simulink model "Propergation_Test"  (R2025b)
settings: Solver=FixedStepAuto  StartTime=0.0  StopTime=inf  RelTol=1e-3
undefined symbols (not defined in the file): bus_b, bus_c
settings Model: SimulationMode=external  Creator=kueh_js  LastModifiedBy=kueh_js
settings OptimizationCC: OptimizeBlockIOStorage=off  EnhancedBackFolding=on  PassReuseOutputArgsThreshold=0.0  ZeroExternalMemoryAtStartup=off  ZeroInternalMemoryAtStartup=off  OptimizeBlockOrder=speed  DifferentSizesBufferReuse=on
settings DebuggingCC: ParameterTunabilityLossMsg=error
settings HardwareCC: ProdBitPerLong=64.0  ProdHWDeviceType=Intel->x86-64 (Linux 64)
settings SFSimCC: MATLABDynamicMemAlloc=off  SimTargetLang=C++  SimDLTargetLibrary=mkl-dnn
settings RTWCC: GenCodeOnly=on  Toolchain=GNU gcc/g++ | gmake (64-bit Linux)  TargetLang=C++
settings CodeAppCC: ForceParamTrailComments=on  OperatorAnnotations=on  MATLABSourceComments=on
settings GRTTargetCC: TargetLangStandard=C++20 (ISO)  MatFileLogging=off  CodeInterfacePackaging=C++ class

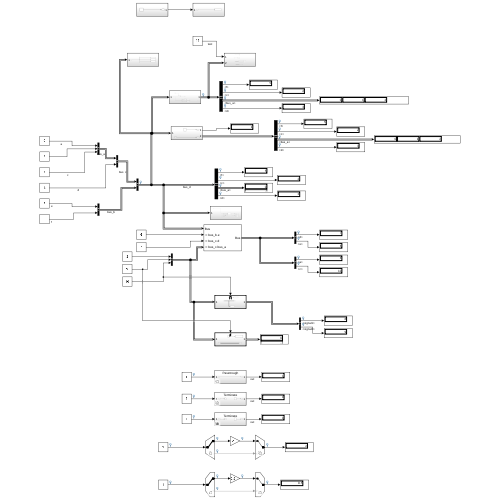
[thumbnail: Simulink's stored preview of the top-level diagram]
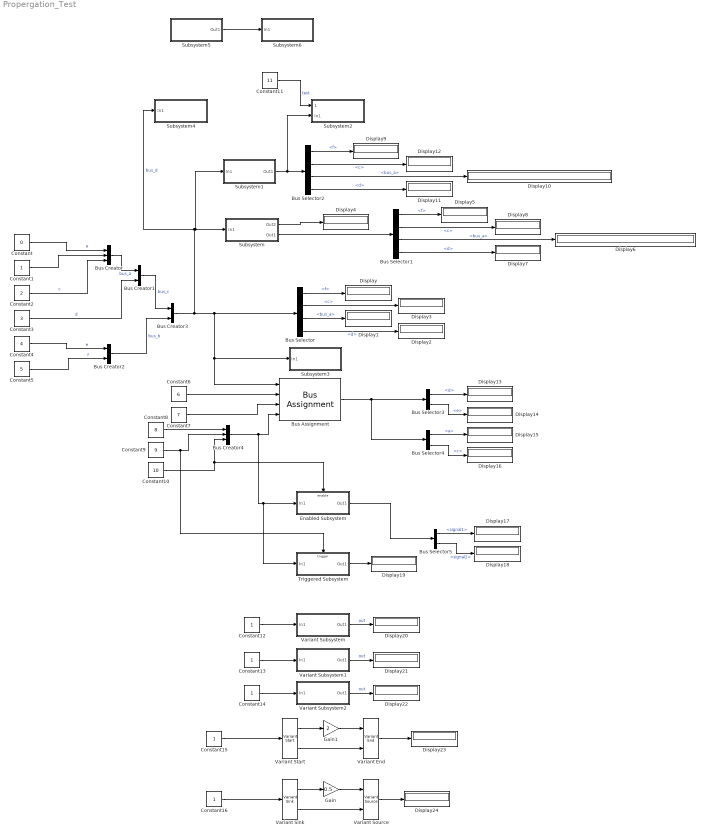
== system Propergation_Test ==
  Bus Assignment : BusAssignment  AssignedSignals=bus_b.e,bus_c.d,bus_c.bus_a
  Bus Creator : BusCreator  Inputs=3
  Bus Creator1 : BusCreator  Inputs=2
  Bus Creator2 : BusCreator  Inputs=2
  Bus Creator3 : BusCreator  Inputs=2
  Bus Creator4 : BusCreator  Inputs=3
  Bus Selector : BusSelector  OutputSignals=bus_b.f,bus_c.bus_a.c,bus_c.bus_a,bus_c.d
  Bus Selector1 : BusSelector  OutputSignals=bus_b.f,bus_c.bus_a.c,bus_c.bus_a,bus_c.d
  Bus Selector2 : BusSelector  OutputSignals=bus_d.bus_b.f,bus_d.bus_c.bus_a.c,bus_d.bus_c.bus_a,bus_d.bus_c.d
  Bus Selector3 : BusSelector  OutputSignals=bus_c.d,bus_b.e
  Bus Selector4 : BusSelector  OutputSignals=bus_c.bus_a.a,bus_c.bus_a.c
  Bus Selector5 : BusSelector  OutputSignals=signal1,signal2
  Constant : Constant  Value=0
  Constant{1,12..16} (6 alike) : Constant
  Constant10 : Constant  Value=10
  Constant11 : Constant  Value=11
  Constant2 : Constant  Value=2
  Constant3 : Constant  Value=3
  Constant4 : Constant  Value=4
  Constant5 : Constant  Value=5
  Constant6 : Constant  Value=6
  Constant7 : Constant  Value=7
  Constant8 : Constant  Value=8
  Constant9 : Constant  Value=9
  Display{,1..24} (25 alike) : Display
  Enabled Subsystem : Subsystem  TreatAsAtomicUnit=on
  Gain : Gain  Gain=0.5
  Gain1 : Gain  Gain=2
  Subsystem : Subsystem
  Subsystem1 : Subsystem
  Subsystem2 : Subsystem
  Subsystem3 : Subsystem
  Subsystem4 : Subsystem
  Subsystem5 : Subsystem
  Subsystem6 : Subsystem
  Triggered Subsystem : Subsystem  TreatAsAtomicUnit=on
  Variant End : VariantEnd
  Variant Sink : VariantSink  VariantControls={true, false}
  Variant Source : VariantSource  VariantControls={true, false}
  Variant Start : VariantStart  VariantControls={true, false}
  Variant Subsystem : Subsystem  Variant=on
  Variant Subsystem1 : Subsystem  Variant=on  VariantControlMode=sim codegen switching
  Variant Subsystem2 : Subsystem  Variant=on  VariantControlMode=label  LabelModeActiveChoice=term
  wires:
  Constant/1 -> Bus Creator/1  "a"
  Constant1/1 -> Bus Creator/2
  Constant2/1 -> Bus Creator/3  "c"
  Bus Creator/1 -> Bus Creator1/1  "bus_a"
  Constant3/1 -> Bus Creator1/2  "d"
  Constant4/1 -> Bus Creator2/1  "e"
  Constant5/1 -> Bus Creator2/2  "f"
  Bus Creator1/1 -> Bus Creator3/1  "bus_c"
  Bus Creator2/1 -> Bus Creator3/2  "bus_b"
  Bus Selector/1 -> Display/1  "<f>"
  Bus Selector/3 -> Display1/1  "<bus_a>"
  Bus Selector/4 -> Display2/1  "<d>"
  Bus Selector/2 -> Display3/1  "<c>"
  Bus Selector1/4 -> Display7/1  "<d>"
  Bus Selector1/1 -> Display5/1  "<f>"
  Subsystem/2(Out1) -> Bus Selector1/1
  Bus Selector1/3 -> Display6/1  "<bus_a>"
  Bus Selector1/2 -> Display8/1  "<c>"
  Bus Selector2/1 -> Display9/1  "<f>"
  Bus Selector2/4 -> Display11/1  "<d>"
  Subsystem1/1(Out1) -> Subsystem2/2(In1), Bus Selector2/1
  Bus Selector2/2 -> Display12/1  "<c>"
  Bus Creator3/1 -> Subsystem4/1(In1), Subsystem1/1(In1), Subsystem/1(In1), Subsystem3/1(In1), Bus Assignment/1, Bus Selector/1  "bus_d"
  Bus Selector2/3 -> Display10/1  "<bus_a>"
  Constant6/1 -> Bus Assignment/2
  Bus Assignment/1 -> Bus Selector4/1, Bus Selector3/1
  Constant7/1 -> Bus Assignment/3
  Bus Selector3/1 -> Display13/1  "<d>"
  Bus Selector3/2 -> Display14/1  "<e>"
  Bus Creator4/1 -> Triggered Subsystem/1(In1), Enabled Subsystem/1(In1), Bus Assignment/4
  Constant8/1 -> Bus Creator4/1
  Constant9/1 -> Triggered Subsystem/Trigger, Bus Creator4/2
  Bus Selector4/1 -> Display15/1  "<a>"
  Bus Selector4/2 -> Display16/1  "<c>"
  Constant10/1 -> Enabled Subsystem/Enable, Bus Creator4/3
  Subsystem/1(Out2) -> Display4/1
  Constant11/1 -> Subsystem2/1(1)  "test"
  Subsystem5/1(Out1) -> Subsystem6/1(In1)
  Bus Selector5/1 -> Display17/1  "<signal1>"
  Enabled Subsystem/1(Out1) -> Bus Selector5/1
  Bus Selector5/2 -> Display18/1  "<signal2>"
  Triggered Subsystem/1(Out1) -> Display19/1
  Constant12/1 -> Variant Subsystem/1(In1)
  Variant Subsystem/1(Out1) -> Display20/1  "out"
  Constant13/1 -> Variant Subsystem1/1(In1)
  Variant Subsystem1/1(Out1) -> Display21/1  "out"
  Variant Subsystem2/1(Out1) -> Display22/1  "out"
  Constant14/1 -> Variant Subsystem2/1(In1)
  Variant Start/2 -> Variant End/2
  Variant Sink/2 -> Variant Source/2
  Gain/1 -> Variant Source/1
  Variant Sink/1 -> Gain/1
  Variant Start/1 -> Gain1/1
  Gain1/1 -> Variant End/1
  Variant End/1 -> Display23/1
  Variant Source/1 -> Display24/1
  Constant15/1 -> Variant Start/1
  Constant16/1 -> Variant Sink/1

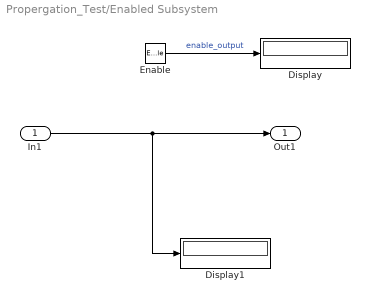
== system Propergation_Test/Enabled Subsystem ==
  In1 : Inport
  Enable : EnablePort  ShowOutputPort=on
  Display : Display
  Display1 : Display
  Out1 : Outport
  wires:
  In1/1 -> Display1/1, Out1/1
  Enable/1 -> Display/1  "enable_output"

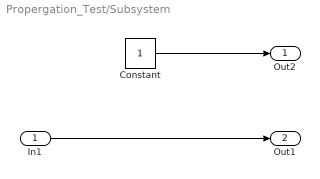
== system Propergation_Test/Subsystem ==
  In1 : Inport
  Constant : Constant
  Out2 : Outport
  Out1 : Outport  Port=2
  wires:
  In1/1 -> Out1/1
  Constant/1 -> Out2/1

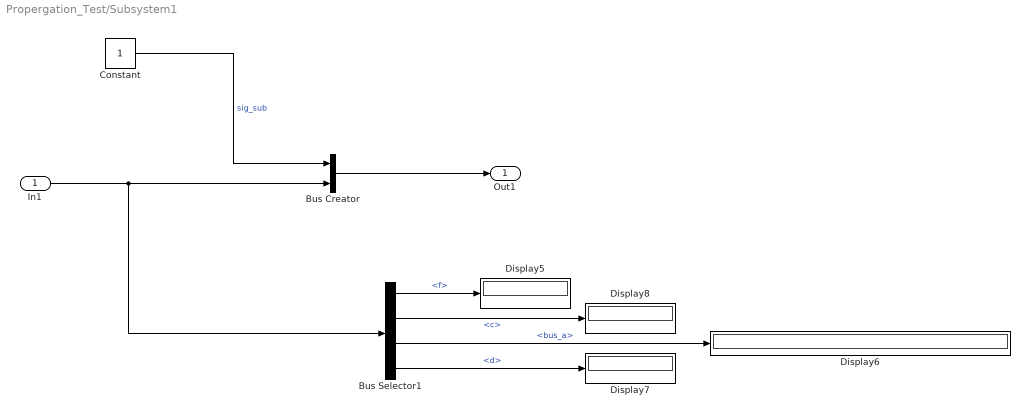
== system Propergation_Test/Subsystem1 ==
  In1 : Inport
  Bus Creator : BusCreator  Inputs=2
  Bus Selector1 : BusSelector  OutputSignals=bus_b.f,bus_c.bus_a.c,bus_c.bus_a,bus_c.d
  Constant : Constant
  Display{5..8} (4 alike) : Display
  Out1 : Outport
  wires:
  Bus Selector1/1 -> Display5/1  "<f>"
  Bus Selector1/4 -> Display7/1  "<d>"
  In1/1 -> Bus Creator/2, Bus Selector1/1
  Bus Selector1/2 -> Display8/1  "<c>"
  Bus Selector1/3 -> Display6/1  "<bus_a>"
  Bus Creator/1 -> Out1/1
  Constant/1 -> Bus Creator/1  "sig_sub"

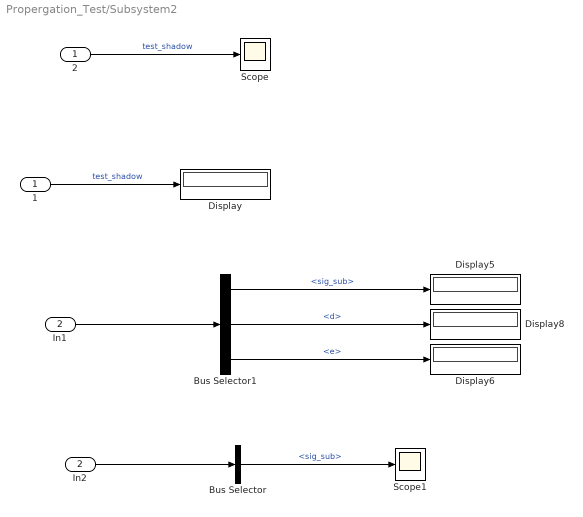
== system Propergation_Test/Subsystem2 ==
  1 : Inport
  In1 : Inport  Port=2
  2 : InportShadow
  Bus Selector : BusSelector  OutputSignals=sig_sub
  Bus Selector1 : BusSelector  OutputSignals=sig_sub,bus_d.bus_c.d,bus_d.bus_b.e
  Display{,5..6,8} (4 alike) : Display
  In2 : InportShadow  Port=2
  Scope : Scope
  Scope1 : Scope
  wires:
  Bus Selector1/1 -> Display5/1  "<sig_sub>"
  In1/1 -> Bus Selector1/1
  Bus Selector1/2 -> Display8/1  "<d>"
  Bus Selector1/3 -> Display6/1  "<e>"
  1/1 -> Display/1  "test_shadow"
  2/1 -> Scope/1  "test_shadow"
  In2/1 -> Bus Selector/1
  Bus Selector/1 -> Scope1/1  "<sig_sub>"

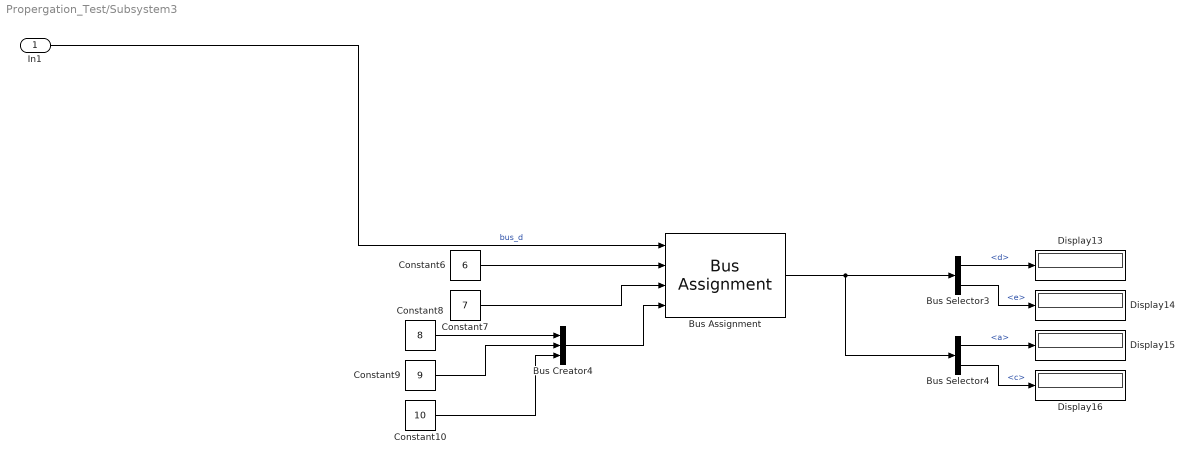
== system Propergation_Test/Subsystem3 ==
  In1 : Inport
  Bus Assignment : BusAssignment  AssignedSignals=bus_b.e,bus_c.d,bus_c.bus_a
  Bus Creator4 : BusCreator  Inputs=3
  Bus Selector3 : BusSelector  OutputSignals=bus_c.d,bus_b.e
  Bus Selector4 : BusSelector  OutputSignals=bus_c.bus_a.a,bus_c.bus_a.c
  Constant10 : Constant  Value=10
  Constant6 : Constant  Value=6
  Constant7 : Constant  Value=7
  Constant8 : Constant  Value=8
  Constant9 : Constant  Value=9
  Display{13..16} (4 alike) : Display
  wires:
  Constant8/1 -> Bus Creator4/1
  Constant9/1 -> Bus Creator4/2
  Bus Selector4/1 -> Display15/1  "<a>"
  Bus Creator4/1 -> Bus Assignment/4
  Constant7/1 -> Bus Assignment/3
  Bus Assignment/1 -> Bus Selector4/1, Bus Selector3/1
  Constant6/1 -> Bus Assignment/2
  Bus Selector4/2 -> Display16/1  "<c>"
  Bus Selector3/2 -> Display14/1  "<e>"
  Bus Selector3/1 -> Display13/1  "<d>"
  In1/1 -> Bus Assignment/1  "bus_d"
  Constant10/1 -> Bus Creator4/3

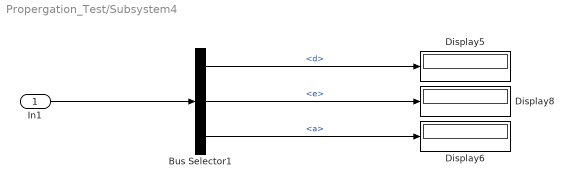
== system Propergation_Test/Subsystem4 ==
  In1 : Inport
  Bus Selector1 : BusSelector  OutputSignals=bus_c.d,bus_b.e,bus_c.bus_a.a
  Display5 : Display
  Display6 : Display
  Display8 : Display
  wires:
  Bus Selector1/1 -> Display5/1  "<d>"
  In1/1 -> Bus Selector1/1
  Bus Selector1/2 -> Display8/1  "<e>"
  Bus Selector1/3 -> Display6/1  "<a>"

== system Propergation_Test/Subsystem5 ==
  Constant : Constant
  Out1 : Outport
  wires:
  Constant/1 -> Out1/1  "test_sub"

== system Propergation_Test/Subsystem6 ==
  In1 : Inport
  Display : Display
  wires:
  In1/1 -> Display/1

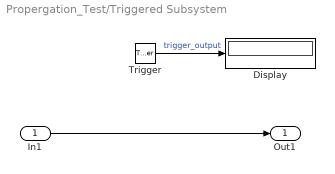
== system Propergation_Test/Triggered Subsystem ==
  In1 : Inport
  Trigger : TriggerPort  VariantControl=(inherit)  ShowOutputPort=on
  Display : Display
  Out1 : Outport
  wires:
  In1/1 -> Out1/1
  Trigger/1 -> Display/1  "trigger_output"

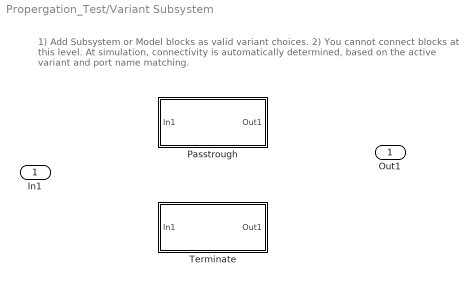
== system Propergation_Test/Variant Subsystem ==
  note: 1) Add Subsystem or Model blocks as valid variant choices.
      | 2) You cannot connect blocks at this level. At simulation, connectivity is automatically
      | determined, based on the active variant and port name matching.
  In1 : Inport
  Passtrough : Subsystem  VariantControl=true
  Terminate : Subsystem  VariantControl=false
  Out1 : Outport

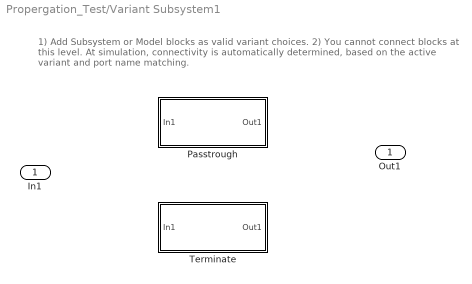
== system Propergation_Test/Variant Subsystem1 ==
  note: 1) Add Subsystem or Model blocks as valid variant choices.
      | 2) You cannot connect blocks at this level. At simulation, connectivity is automatically
      | determined, based on the active variant and port name matching.
  In1 : Inport
  Passtrough : Subsystem  VariantControl=(codegen)
  Terminate : Subsystem  VariantControl=(sim)
  Out1 : Outport

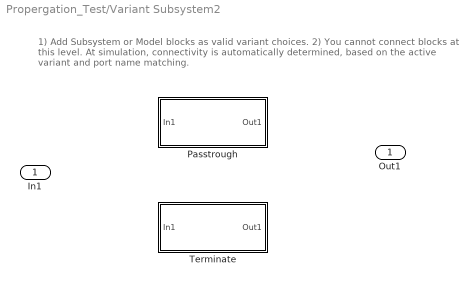
== system Propergation_Test/Variant Subsystem2 ==
  note: 1) Add Subsystem or Model blocks as valid variant choices.
      | 2) You cannot connect blocks at this level. At simulation, connectivity is automatically
      | determined, based on the active variant and port name matching.
  In1 : Inport
  Passtrough : Subsystem  VariantControl=pass
  Terminate : Subsystem  VariantControl=term
  Out1 : Outport

== system Propergation_Test/Variant Subsystem/Passtrough ==
  In1 : Inport
  Out1 : Outport
  wires:
  In1/1 -> Out1/1

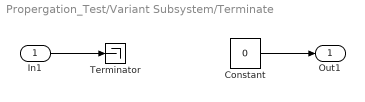
== system Propergation_Test/Variant Subsystem/Terminate ==
  In1 : Inport
  Constant : Constant  Value=0
  Terminator : Terminator
  Out1 : Outport
  wires:
  In1/1 -> Terminator/1
  Constant/1 -> Out1/1

== system Propergation_Test/Variant Subsystem1/Passtrough ==
  In1 : Inport
  Out1 : Outport
  wires:
  In1/1 -> Out1/1

== system Propergation_Test/Variant Subsystem1/Terminate ==
  In1 : Inport
  Constant : Constant  Value=0
  Terminator : Terminator
  Out1 : Outport
  wires:
  In1/1 -> Terminator/1
  Constant/1 -> Out1/1

== system Propergation_Test/Variant Subsystem2/Passtrough ==
  In1 : Inport
  Out1 : Outport
  wires:
  In1/1 -> Out1/1

== system Propergation_Test/Variant Subsystem2/Terminate ==
  In1 : Inport
  Constant : Constant  Value=0
  Terminator : Terminator
  Out1 : Outport
  wires:
  In1/1 -> Terminator/1
  Constant/1 -> Out1/1
